simulink model "circle_MAfilt_post"  (R2024b)
settings: Solver=VariableStepAuto  StartTime=0.0  StopTime=7  RelTol=1e-3
values from neighbouring files (symbols this model uses):
  Rc = 1    [calc_circler_interpolation.m]    (also in load_params.m)
  tau = 1    [calc_circler_interpolation.m]    (also in load_params.m)
  wc = 1    [calc_circler_interpolation.m]    (also in load_params.m)
settings Model: Creator=shohei  LastModifiedBy=shohei

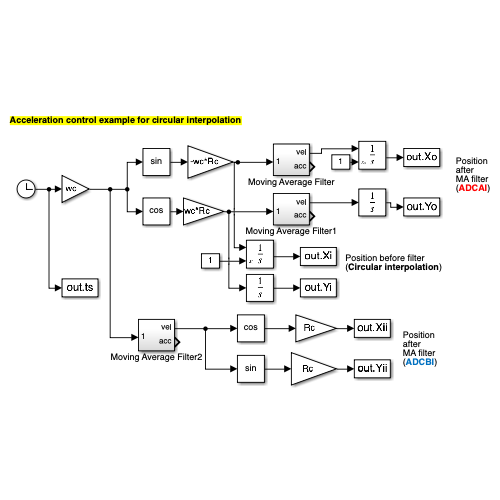
[thumbnail: Simulink's stored preview of the top-level diagram]
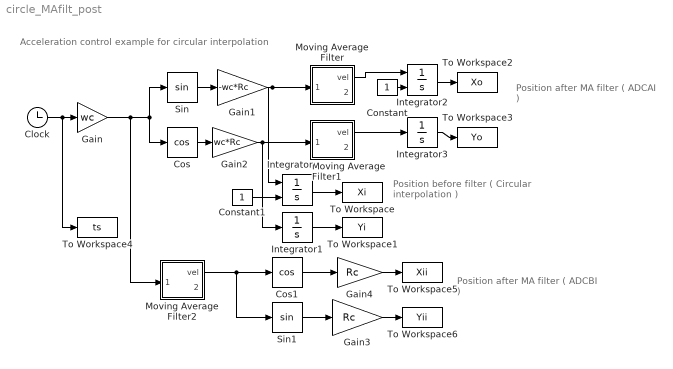
== system circle_MAfilt_post ==
  note: Acceleration control example for circular interpolation
  note: Position before filter
      | ( Circular interpolation )
  note: Position
      | after
      | MA filter
      | ( ADCAI )
  note: Position
      | after
      | MA filter
      | ( ADCBI )
  Clock : Clock
  Constant : Constant
  Constant1 : Constant
  Cos : Trigonometry  Operator=cos
  Cos1 : Trigonometry  Operator=cos
  Gain : Gain  Gain=wc
  Gain1 : Gain  Gain=-wc*Rc
  Gain2 : Gain  Gain=wc*Rc
  Gain3 : Gain  Gain=Rc
  Gain4 : Gain  Gain=Rc
  Integrator : Integrator  InitialConditionSource=external  InitialCondition=1
  Integrator1 : Integrator
  Integrator2 : Integrator  InitialConditionSource=external  InitialCondition=1
  Integrator3 : Integrator
  Moving Average Filter : Subsystem
  Moving Average Filter1 : Subsystem
  Moving Average Filter2 : Subsystem
  Sin : Trigonometry
  Sin1 : Trigonometry
  To Workspace : ToWorkspace  VariableName=Xi  SaveFormat=Timeseries  SampleTime=-1
  To Workspace1 : ToWorkspace  VariableName=Yi  SaveFormat=Timeseries  SampleTime=-1
  To Workspace2 : ToWorkspace  VariableName=Xo  SaveFormat=Timeseries  SampleTime=-1
  To Workspace3 : ToWorkspace  VariableName=Yo  SaveFormat=Timeseries  SampleTime=-1
  To Workspace4 : ToWorkspace  VariableName=ts  SaveFormat=Timeseries  SampleTime=-1
  To Workspace5 : ToWorkspace  VariableName=Xii  SaveFormat=Timeseries  SampleTime=-1
  To Workspace6 : ToWorkspace  VariableName=Yii  SaveFormat=Timeseries  SampleTime=-1
  wires:
  Clock/1 -> To Workspace4/1, Gain/1
  Sin/1 -> Gain1/1
  Cos/1 -> Gain2/1
  Gain/1 -> Moving Average Filter2/1(In1), Sin/1, Cos/1
  Gain1/1 -> Integrator/1, Moving Average Filter/1(In1)
  Integrator/1 -> To Workspace/1
  Integrator1/1 -> To Workspace1/1
  Moving Average Filter/1(vel) -> Integrator2/1
  Integrator2/1 -> To Workspace2/1
  Gain2/1 -> Integrator1/1, Moving Average Filter1/1(In1)
  Integrator3/1 -> To Workspace3/1
  Moving Average Filter1/1(vel) -> Integrator3/1
  Gain3/1 -> To Workspace6/1
  Gain4/1 -> To Workspace5/1
  Cos1/1 -> Gain4/1
  Sin1/1 -> Gain3/1
  Moving Average Filter2/1(vel) -> Sin1/1, Cos1/1
  Constant/1 -> Integrator2/2
  Constant1/1 -> Integrator/2

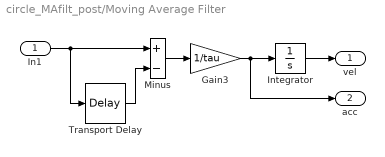
== system circle_MAfilt_post/Moving Average Filter ==
  In1 : Inport
  Gain3 : Gain  Gain=1/tau
  Integrator : Integrator
  Minus : Sum  Inputs=+-
  Transport Delay : TransportDelay  DelayTime=tau
  vel : Outport
  acc : Outport  Port=2
  wires:
  In1/1 -> Minus/1, Transport Delay/1
  Integrator/1 -> vel/1
  Gain3/1 -> acc/1, Integrator/1
  Transport Delay/1 -> Minus/2
  Minus/1 -> Gain3/1

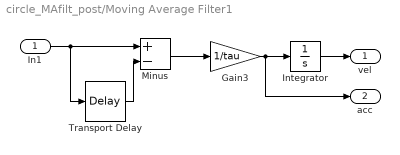
== system circle_MAfilt_post/Moving Average Filter1 ==
  In1 : Inport
  Gain3 : Gain  Gain=1/tau
  Integrator : Integrator
  Minus : Sum  Inputs=+-
  Transport Delay : TransportDelay  DelayTime=tau
  vel : Outport
  acc : Outport  Port=2
  wires:
  In1/1 -> Minus/1, Transport Delay/1
  Integrator/1 -> vel/1
  Gain3/1 -> acc/1, Integrator/1
  Transport Delay/1 -> Minus/2
  Minus/1 -> Gain3/1

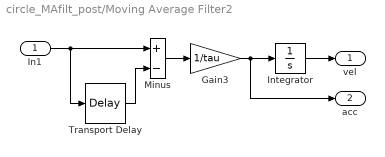
== system circle_MAfilt_post/Moving Average Filter2 ==
  In1 : Inport
  Gain3 : Gain  Gain=1/tau
  Integrator : Integrator
  Minus : Sum  Inputs=+-
  Transport Delay : TransportDelay  DelayTime=tau
  vel : Outport
  acc : Outport  Port=2
  wires:
  In1/1 -> Minus/1, Transport Delay/1
  Integrator/1 -> vel/1
  Gain3/1 -> acc/1, Integrator/1
  Transport Delay/1 -> Minus/2
  Minus/1 -> Gain3/1
